simulink model "rgb_arduino3"  (R2019b)
settings: Solver=FixedStepDiscrete  StartTime=0.0  StopTime=10.0  FixedStep=0.01  RelTol=1e-3
libraries: arduinolib x6
settings Model: ExtModeTrigDuration=2  Creator=roslovetspv  LastModifiedBy=bhisma
settings DataIOCC: ReturnWorkspaceOutputs=off
settings OptimizationCC: LifeSpan=1  MaxStackSize=64  EfficientTunableParamExpr=on
settings DebuggingCC: SFUnexpectedBacktrackingDiag=warning  SFNoUnconditionalDefaultTransitionDiag=warning  ArithmeticOperatorsInVariantConditions=warning
settings HardwareCC: ProdBitPerInt=16  ProdBitPerPointer=16  ProdBitPerSizeT=16  ProdBitPerPtrDiffT=16  ProdLargestAtomicFloat=None  ProdWordSize=8  ProdHWDeviceType=Atmel->AVR
settings SFSimCC: SimUseLocalCustomCode=off  MATLABDynamicMemAlloc=off  CustomCodeUndefinedFunction=UseInterfaceOnly
settings RTWCC: SystemTargetFile=ert.tlc  HardwareBoard=Arduino Uno  TLCOptions=-aInlineSetEventsForThisBaseRateFcn=TLC_FALSE -aSuppressMultiTaskScheduler=TLC_FALSE -aRateBasedStepFcn=1  TemplateMakefile=ert_default_tmf  GenerateReport=on  RTWUseLocalCustomCode=off  Toolchain=Arduino AVR v1.6.1  BuildConfiguration=Faster Runs  IncludeHyperlinkInReport=on  LaunchReport=on  GenerateTraceInfo=on  GenerateTraceReport=on  GenerateTraceReportSl=on  GenerateTraceReportSf=on  GenerateTraceReportEml=on
settings CodeAppCC: ForceParamTrailComments=on  IgnoreCustomStorageClasses=off  OperatorAnnotations=on  SimulinkDataObjDesc=on  SFDataObjDesc=on  MATLABFcnDesc=on  InsertBlockDesc=on  StateflowObjectComments=on  MATLABSourceComments=on
settings ERTTargetCC: MultiwordLength=2048  SupportContinuousTime=on  SupportVariableSizeSignals=on
settings ConfigComp: CovMetricSettings=dw  CovHtmlReporting=on  CovSaveCumulativeToWorkspaceVar=on  CovSaveSingleToWorkspaceVar=on  CovExternalEMLEnable=off
settings SimscapeCC: SimscapeNormalizeSystem=off

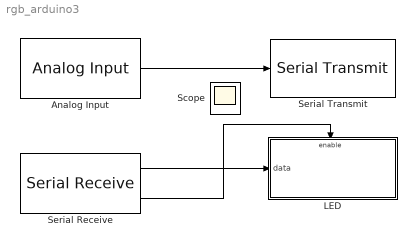
== system rgb_arduino3 ==
  Analog Input : arduinolib/Analog Input  pinNumber=0  sampleTime=0.07  blockPlatform=arduino
  LED : Subsystem  TreatAsAtomicUnit=on
  Serial Receive : arduinolib/Serial Receive  portNumber=0  showOutStatus=on  sampleTime=0.01  blockPlatform=arduino
      settings: SourceProductName=Simulink Support Package for Arduino Hardware  SourceProductBaseCode=ARDUINO
  Serial Transmit : arduinolib/Serial Transmit  portNumber=0  blockPlatform=arduino
      settings: SourceProductName=Simulink Support Package for Arduino Hardware
  Scope : Scope
  wires:
  Serial Receive/2 -> LED/Enable
  Serial Receive/1 -> LED/1(data)
  Analog Input/1 -> Serial Transmit/1

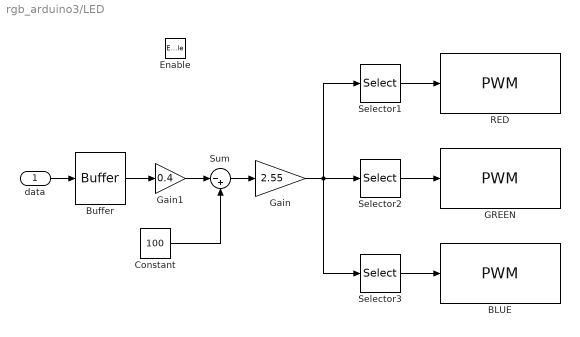
== system rgb_arduino3/LED ==
  data : Inport
  Enable : EnablePort
  BLUE : arduinolib/PWM  pinNumber=11  blockPlatform=arduino
  Buffer : Buffer  N=3  OutputFrames=off
  Constant : Constant  Value=100
  GREEN : arduinolib/PWM  pinNumber=10  blockPlatform=arduino
  Gain : Gain  Gain=2.55
  Gain1 : Gain  Gain=0.4
  RED : arduinolib/PWM  pinNumber=9  blockPlatform=arduino
  Selector1 : Selector  InputPortWidth=3  IndexOptions=Index vector (dialog)  Indices=1  OutputSizes=1
  Selector2 : Selector  InputPortWidth=3  IndexOptions=Index vector (dialog)  Indices=2  OutputSizes=1
  Selector3 : Selector  InputPortWidth=3  IndexOptions=Index vector (dialog)  Indices=3  OutputSizes=1
  Sum : Sum  Inputs=|-+
  wires:
  data/1 -> Buffer/1
  Sum/1 -> Gain/1
  Selector2/1 -> GREEN/1
  Selector3/1 -> BLUE/1
  Selector1/1 -> RED/1
  Buffer/1 -> Gain1/1
  Constant/1 -> Sum/2
  Gain/1 -> Selector1/1, Selector2/1, Selector3/1
  Gain1/1 -> Sum/1
